simulink model "asbQuadcopters_SiFi"  (Simulink 9.1)
settings: Solver=VariableStepAuto  StartTime=0.0  StopTime=TFinal  RelTol=1e-3
values from neighbouring files (symbols this model uses):
  Controller =     [data_set.mat]
  Estimator =     [data_set.mat]
  g = 9.81    [data_set.mat]
  init =     [data_set.mat]
  rho = 1.184    [data_set.mat]
  sensorCalibrationData = [0.09 -0.06 -9.473 -0.0095 -0.0075 0.0015 101270.95 0.2]    [data_set.mat]
  Sensors =     [data_set.mat]
  States =     [data_set.mat]
  takeOffDuration = 1    [data_set.mat]
  Ts = 0.005    [data_set.mat]
  Vehicle =     [data_set.mat]
undefined symbols (not defined in the file or in its folder): DiscIntNeverNeededParam, Discrete, Earth, ft, m, s, sigbuilder_block, Time, WGS84
libraries: F_Line_block x565, simulink x39, aerolibconvert2 x4, sharedutil x3, ctrlSharedLib x3, sharedtransform x3, shared6dof x1, aerolibasang x1, aerolibtransform2 x1, aerolibnav x1, aerolibanimutils x1
(part 2 of 4)

== system asbQuadcopters_SiFi/Airframe/AC model/Gravity Force Calculation ==
  DCMbe : Inport
  gravity : Inport  Port=2  Unit=m/s^2
  Gain1 : Gain  Gain=Vehicle.Airframe.mass
  FAULT_Gain1 : F_Line_block/Subsystem
  Product : Product  Multiplication=Matrix(*)
  FAULT_Product : F_Line_block/Subsystem
  FAULT_Product_2 : F_Line_block/Subsystem
  gravity force : Outport  Unit=N
  FAULT_gravity force : F_Line_block/Subsystem
  wires:
  gravity/1 -> FAULT_Gain1/1
  FAULT_Gain1/1 -> Gain1/1
  Gain1/1 -> FAULT_Product_2/1  "gravity force NED"
  FAULT_Product_2/1 -> Product/2
  Product/1 -> FAULT_gravity force/1
  FAULT_gravity force/1 -> gravity force/1
  DCMbe/1 -> FAULT_Product/1
  FAULT_Product/1 -> Product/1

== system asbQuadcopters_SiFi/Airframe/AC model/Motor Forces and Torques ==
  Vb : Inport
  Density : Inport  Port=2
  pqr : Inport  Port=3
  Motor  Commands : Inport  Port=4
  D1 : Constant  Value=[Vehicle.Airframe.xy -Vehicle.Airframe.xy Vehicle.Airframe.h]
  D2 : Constant  Value=[Vehicle.Airframe.xy Vehicle.Airframe.xy Vehicle.Airframe.h]
  D3 : Constant  Value=[-Vehicle.Airframe.xy Vehicle.Airframe.xy Vehicle.Airframe.h]
  D4 : Constant  Value=[-Vehicle.Airframe.xy -Vehicle.Airframe.xy Vehicle.Airframe.h]
  For Each Subsystem : Subsystem
  MotorsToW : Subsystem
  Sum of Elements : Sum  Inputs=+  CollapseMode=Specified dimension  CollapseDim=2
  FAULT_Sum of Elements : F_Line_block/Subsystem
  Sum of Elements1 : Sum  Inputs=+  CollapseMode=Specified dimension  CollapseDim=2
  FAULT_Sum of Elements1 : F_Line_block/Subsystem
  Vector Concatenate : Concatenate  NumInputs=4  Mode=Multidimensional array  ConcatenateDimension=2
  FAULT_Vector Concatenate : F_Line_block/Subsystem
  FAULT_Vector Concatenate_2 : F_Line_block/Subsystem
  FAULT_Vector Concatenate_3 : F_Line_block/Subsystem
  FAULT_Vector Concatenate_4 : F_Line_block/Subsystem
  Motor Forces : Outport  Unit=N
  FAULT_Motor Forces : F_Line_block/Subsystem
  Motor Torques : Outport  Port=2  Unit=N*m
  FAULT_Motor Torques : F_Line_block/Subsystem
  wires:
  D2/1 -> FAULT_Vector Concatenate_2/1
  FAULT_Vector Concatenate_2/1 -> Vector Concatenate/2
  D3/1 -> FAULT_Vector Concatenate_3/1
  FAULT_Vector Concatenate_3/1 -> Vector Concatenate/3
  D1/1 -> FAULT_Vector Concatenate/1
  FAULT_Vector Concatenate/1 -> Vector Concatenate/1
  Vector Concatenate/1 -> For Each Subsystem/5(D)
  pqr/1 -> For Each Subsystem/3(Omega)
  For Each Subsystem/2(Moments) -> FAULT_Sum of Elements1/1
  FAULT_Sum of Elements1/1 -> Sum of Elements1/1
  Sum of Elements/1 -> FAULT_Motor Forces/1
  FAULT_Motor Forces/1 -> Motor Forces/1
  Vb/1 -> For Each Subsystem/1(Vb)
  Motor  Commands/1 -> MotorsToW/1(motors_datin)
  For Each Subsystem/1(Forces) -> FAULT_Sum of Elements/1
  FAULT_Sum of Elements/1 -> Sum of Elements/1
  MotorsToW/1(omegas_datout) -> For Each Subsystem/4(w)
  D4/1 -> FAULT_Vector Concatenate_4/1
  FAULT_Vector Concatenate_4/1 -> Vector Concatenate/4
  Density/1 -> For Each Subsystem/2(rho)
  Sum of Elements1/1 -> FAULT_Motor Torques/1
  FAULT_Motor Torques/1 -> Motor Torques/1

== system asbQuadcopters_SiFi/FCS/Crash Predictor Flags/Geofencing error ==
  Action Port : ActionPort  ActionType=then
  FAULT_Action Port : F_Line_block/Subsystem
  Constant : Constant  OutDataTypeStr=uint8
  Out1 : Outport
  FAULT_Out1 : F_Line_block/Subsystem
  wires:
  Constant/1 -> FAULT_Out1/1
  FAULT_Out1/1 -> Out1/1

== system asbQuadcopters_SiFi/FCS/Crash Predictor Flags/Normal condition ==
  Action Port : ActionPort  ActionType=else
  FAULT_Action Port : F_Line_block/Subsystem
  Constant : Constant  Value=0  OutDataTypeStr=uint8
  Out1 : Outport
  FAULT_Out1 : F_Line_block/Subsystem
  wires:
  Constant/1 -> FAULT_Out1/1
  FAULT_Out1/1 -> Out1/1

== system asbQuadcopters_SiFi/FCS/Crash Predictor Flags/estimator/Optical flow error ==
  Action Port : ActionPort  ActionType=elseif
  FAULT_Action Port : F_Line_block/Subsystem
  Constant : Constant  Value=99  OutDataTypeStr=uint8
  Out1 : Outport
  FAULT_Out1 : F_Line_block/Subsystem
  wires:
  Constant/1 -> FAULT_Out1/1
  FAULT_Out1/1 -> Out1/1

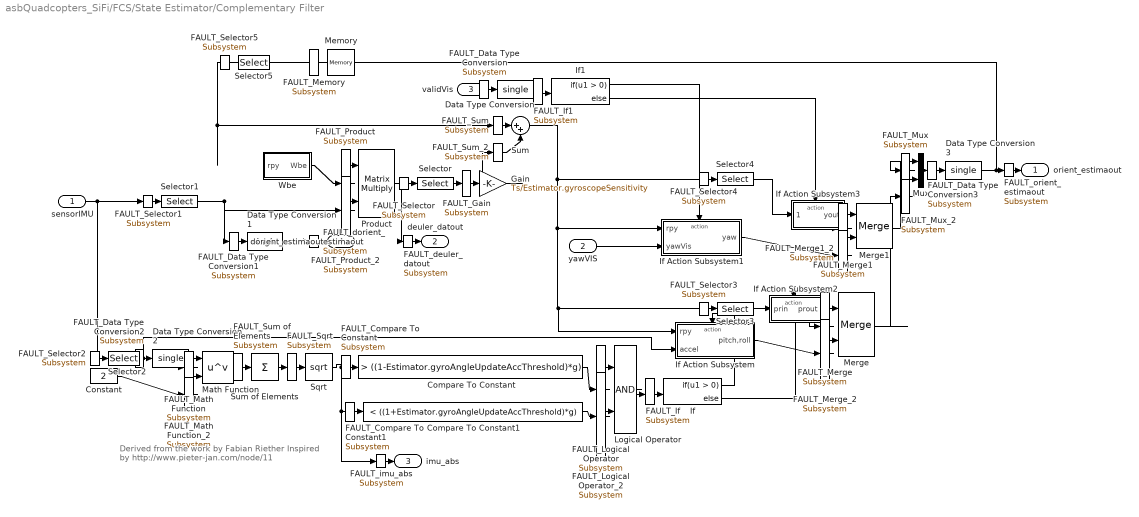
== system asbQuadcopters_SiFi/FCS/State Estimator/Complementary Filter ==
  note: Derived from the work by Fabian Riether
      | Inspired by http://www.pieter-jan.com/node/11
  sensorIMU : Inport  OutDataTypeStr=single
  yawVIS : Inport  Port=2
  validVis : Inport  Port=3
  Compare To Constant : simulink/Logic and Bit Operations/Compare To Constant  relop=>  const=((1-Estimator.gyroAngleUpdateAccThreshold)*g)  OutDataTypeStr=boolean
  FAULT_Compare To Constant : F_Line_block/Subsystem
  Compare To Constant1 : simulink/Logic and Bit Operations/Compare To Constant  relop=<  const=((1+Estimator.gyroAngleUpdateAccThreshold)*g)  OutDataTypeStr=boolean
  FAULT_Compare To Constant1 : F_Line_block/Subsystem
  Constant : Constant  Value=2  OutDataTypeStr=single
  Data Type Conversion{,1..3} (4 alike) : DataTypeConversion  OutDataTypeStr=single
  FAULT_Data Type Conversion{,1..3} (4 alike) : F_Line_block/Subsystem
  Gain : Gain  Gain=Ts/Estimator.gyroscopeSensitivity
  FAULT_Gain : F_Line_block/Subsystem
  If : If
  FAULT_If : F_Line_block/Subsystem
  If Action Subsystem : Subsystem  TreatAsAtomicUnit=on
  If Action Subsystem1 : Subsystem  TreatAsAtomicUnit=on
  If Action Subsystem2 : Subsystem  TreatAsAtomicUnit=on
  If Action Subsystem3 : Subsystem  TreatAsAtomicUnit=on
  If1 : If
  FAULT_If1 : F_Line_block/Subsystem
  Logical Operator : Logic  AllPortsSameDT=off  OutDataTypeStr=fixdt(1,16)
  FAULT_Logical Operator : F_Line_block/Subsystem
  FAULT_Logical Operator_2 : F_Line_block/Subsystem
  Math Function : Math  Operator=pow  SaturateOnIntegerOverflow=on
  FAULT_Math Function : F_Line_block/Subsystem
  FAULT_Math Function_2 : F_Line_block/Subsystem
  Memory : Memory  InitialCondition=single(Estimator.complementaryFilterInit)  InheritSampleTime=on
  FAULT_Memory : F_Line_block/Subsystem
  Merge : Merge
  FAULT_Merge : F_Line_block/Subsystem
  FAULT_Merge_2 : F_Line_block/Subsystem
  Merge1 : Merge
  FAULT_Merge1 : F_Line_block/Subsystem
  FAULT_Merge1_2 : F_Line_block/Subsystem
  Mux : Mux  Inputs=2
  FAULT_Mux : F_Line_block/Subsystem
  FAULT_Mux_2 : F_Line_block/Subsystem
  Product : Product  Multiplication=Matrix(*)
  FAULT_Product : F_Line_block/Subsystem
  FAULT_Product_2 : F_Line_block/Subsystem
  Selector : Selector  InputPortWidth=3  IndexOptions=Index vector (dialog)  Indices=[3 2 1]  OutputSizes=1
  FAULT_Selector{,1..5} (6 alike) : F_Line_block/Subsystem
  Selector1 : Selector  InputPortWidth=6  IndexOptions=Index vector (dialog)  Indices=[4 5 6]  OutputSizes=1
  Selector2 : Selector  InputPortWidth=6  IndexOptions=Index vector (dialog)  Indices=[1 2 3]  OutputSizes=1
  Selector3 : Selector  InputPortWidth=3  IndexOptions=Index vector (dialog)  Indices=[2 1]  OutputSizes=1
  Selector4 : Selector  InputPortWidth=3  IndexOptions=Index vector (dialog)  Indices=[3]  OutputSizes=1
  Selector5 : Selector  InputPortWidth=3  IndexOptions=Index vector (dialog)  Indices=[3 2 1]  OutputSizes=1
  Sqrt : Sqrt  SaturateOnIntegerOverflow=on
  FAULT_Sqrt : F_Line_block/Subsystem
  Sum : Sum  Inputs=|++
  FAULT_Sum : F_Line_block/Subsystem
  FAULT_Sum_2 : F_Line_block/Subsystem
  Sum of Elements : Sum  Inputs=+
  FAULT_Sum of Elements : F_Line_block/Subsystem
  Wbe : Subsystem
  orient_estimaout : Outport
  FAULT_orient_estimaout : F_Line_block/Subsystem
  deuler_datout : Outport  Port=2
  FAULT_deuler_datout : F_Line_block/Subsystem
  imu_abs : Outport  Port=3  OutDataTypeStr=single
  FAULT_imu_abs : F_Line_block/Subsystem
  dorient_estimaout : Outport  Port=4
  FAULT_dorient_estimaout : F_Line_block/Subsystem
  wires:
  sensorIMU/1 -> FAULT_Selector1/1, FAULT_Selector2/1
  FAULT_Selector1/1 -> Selector1/1
  FAULT_Selector2/1 -> Selector2/1
  Product/1 -> FAULT_deuler_datout/1, FAULT_Selector/1
  FAULT_deuler_datout/1 -> deuler_datout/1
  FAULT_Selector/1 -> Selector/1
  Wbe/1(Wbe) -> FAULT_Product/1
  FAULT_Product/1 -> Product/1
  Selector/1 -> FAULT_Gain/1
  FAULT_Gain/1 -> Gain/1
  Gain/1 -> FAULT_Sum_2/1
  FAULT_Sum_2/1 -> Sum/2
  Memory/1 -> FAULT_Selector5/1
  FAULT_Selector5/1 -> Selector5/1
  Sum of Elements/1 -> FAULT_Sqrt/1
  FAULT_Sqrt/1 -> Sqrt/1
  Math Function/1 -> FAULT_Sum of Elements/1
  FAULT_Sum of Elements/1 -> Sum of Elements/1
  Constant/1 -> FAULT_Math Function_2/1
  FAULT_Math Function_2/1 -> Math Function/2
  Selector2/1 -> If Action Subsystem/2(accel), FAULT_Data Type Conversion2/1
  FAULT_deuler_datout/1 -> deuler_datout/1
  FAULT_Data Type Conversion2/1 -> Data Type Conversion2/1
  Sqrt/1 -> FAULT_imu_abs/1, Compare To Constant1/1, Compare To Constant/1
  Compare To Constant/1 -> FAULT_Logical Operator/1
  FAULT_Logical Operator/1 -> Logical Operator/1
  Compare To Constant1/1 -> FAULT_Logical Operator_2/1
  FAULT_Logical Operator_2/1 -> Logical Operator/2
  If Action Subsystem/1(pitch,roll) -> FAULT_Merge_2/1
  FAULT_Merge_2/1 -> Merge/2
  Sum/1 -> If Action Subsystem1/1(rpy), If Action Subsystem/1(rpy), Selector3/1, Selector4/1
  Selector3/1 -> If Action Subsystem2/1(prin)
  yawVIS/1 -> If Action Subsystem1/2(yawVis)
  Selector4/1 -> If Action Subsystem3/1(yawin)
  If Action Subsystem1/1(yaw) -> FAULT_Merge1_2/1
  FAULT_imu_abs/1 -> imu_abs/1
  FAULT_Data Type Conversion2/1 -> Data Type Conversion2/1
  FAULT_Selector2/1 -> Selector2/1
  FAULT_Merge1_2/1 -> Merge1/2
  Merge/1 -> FAULT_Mux_2/1
  FAULT_Mux_2/1 -> Mux/2
  Mux/1 -> FAULT_Data Type Conversion3/1
  FAULT_Data Type Conversion3/1 -> Data Type Conversion3/1
  If Action Subsystem2/1(prout) -> FAULT_Merge/1
  FAULT_Merge/1 -> Merge/1
  If/2 -> If Action Subsystem2/Action
  If Action Subsystem3/1(yout) -> FAULT_Merge1/1
  FAULT_Merge1/1 -> Merge1/1
  If1/2 -> If Action Subsystem3/Action
  Logical Operator/1 -> FAULT_If/1
  FAULT_If/1 -> If/1
  If/1 -> If Action Subsystem/Action
  If1/1 -> If Action Subsystem1/Action
  Data Type Conversion/1 -> FAULT_If1/1
  FAULT_If1/1 -> If1/1
  validVis/1 -> FAULT_Data Type Conversion/1
  FAULT_Data Type Conversion/1 -> Data Type Conversion/1
  Selector1/1 -> FAULT_Product_2/1, FAULT_Data Type Conversion1/1
  FAULT_Product_2/1 -> Product/2
  FAULT_Data Type Conversion1/1 -> Data Type Conversion1/1
  Data Type Conversion2/1 -> FAULT_Math Function/1
  FAULT_Math Function/1 -> Math Function/1
  Data Type Conversion3/1 -> FAULT_Memory/1, FAULT_orient_estimaout/1
  FAULT_Memory/1 -> Memory/1
  FAULT_orient_estimaout/1 -> orient_estimaout/1
  Merge1/1 -> FAULT_Mux/1
  FAULT_Mux/1 -> Mux/1
  Selector5/1 -> FAULT_Sum/1, ?FAULT_Wbe/1
  FAULT_Sum/1 -> Sum/1
  ?FAULT_Wbe/1 -> Wbe/1(rpy)
  Data Type Conversion1/1 -> FAULT_dorient_estimaout/1
  FAULT_dorient_estimaout/1 -> dorient_estimaout/1

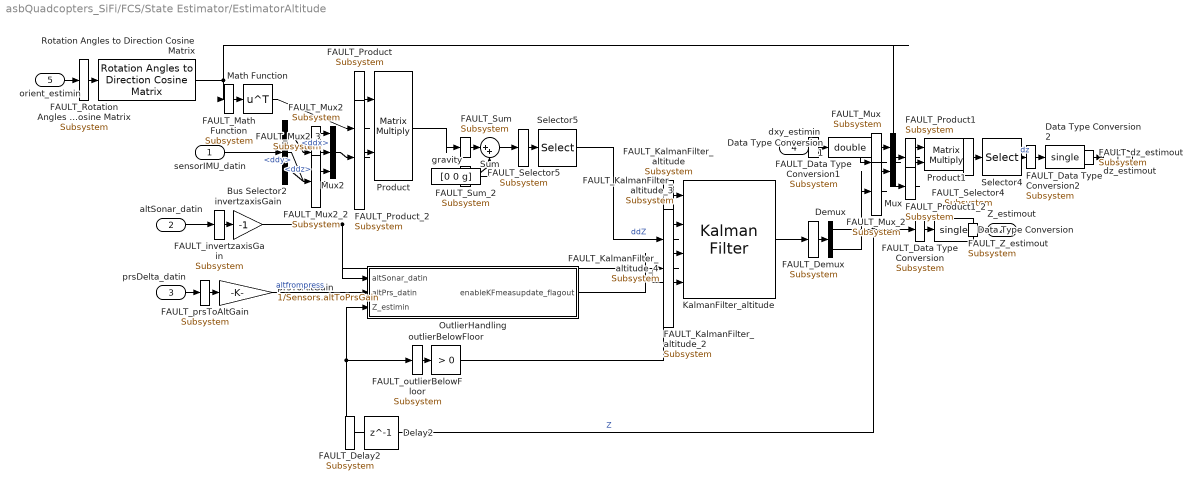
== system asbQuadcopters_SiFi/FCS/State Estimator/EstimatorAltitude ==
  sensorIMU_datin : Inport
  altSonar_datin : Inport  Port=2
  prsDelta_datin : Inport  Port=3
  dxy_estimin : Inport  Port=4
  orient_estimin : Inport  Port=5
  Bus Selector2 : BusSelector  OutputSignals=ddx,ddy,ddz
  Data Type Conversion : DataTypeConversion  OutDataTypeStr=single  SaturateOnIntegerOverflow=on
  FAULT_Data Type Conversion : F_Line_block/Subsystem
  Data Type Conversion1 : DataTypeConversion  OutDataTypeStr=double  SaturateOnIntegerOverflow=on
  FAULT_Data Type Conversion1 : F_Line_block/Subsystem
  Data Type Conversion2 : DataTypeConversion  OutDataTypeStr=single  SaturateOnIntegerOverflow=on
  FAULT_Data Type Conversion2 : F_Line_block/Subsystem
  Delay2 : Delay  DelayLength=1  InitialCondition=0
  FAULT_Delay2 : F_Line_block/Subsystem
  Demux : Demux  Outputs=2
  FAULT_Demux : F_Line_block/Subsystem
  KalmanFilter_altitude : ctrlSharedLib/Kalman Filter  TimeDomain=Discrete-Time  UseCurrentEstimator=on  ModelSource=Individual A, B, C, D matrices  ModelSourceVariable=sys  A=[1 Ts; 0 1]  B=[0;Ts]  C=[1 0]  D=[0]  NumberOfStates=2  NumberOfInputs=2  NumberOfOutputs=2  InitialEstimateSource=Dialog  X0=[init.posNED(3) 0]  P0=10  UseK=off  UseGH=on  NumberOfProcessNoiseInputs=2  G=Estimator.alt.kf.G  TimeInvariantG=on  H=Estimator.alt.kf.H  TimeInvariantH=on  Q=Estimator.alt.kf.Q  TimeInvariantQ=on  R=Estimator.alt.kf.R  TimeInvariantR=on  N=Estimator.alt.kf.N  TimeInvariantN=on  AddInputPort=on  AddEnablePort=on  ExternalReset=Level hold  OutputEstimatedY=off  OutputP=off  Ts=-1
      settings: SourceProductBaseCode=CT
  FAULT_KalmanFilter_altitude : F_Line_block/Subsystem
  FAULT_KalmanFilter_altitude_2 : F_Line_block/Subsystem
  FAULT_KalmanFilter_altitude_3 : F_Line_block/Subsystem
  FAULT_KalmanFilter_altitude_4 : F_Line_block/Subsystem
  Math Function : Math  Operator=transpose  SaturateOnIntegerOverflow=on
  FAULT_Math Function : F_Line_block/Subsystem
  Mux : Mux  Inputs=2
  FAULT_Mux : F_Line_block/Subsystem
  FAULT_Mux_2 : F_Line_block/Subsystem
  Mux2 : Mux  Inputs=3
  FAULT_Mux2 : F_Line_block/Subsystem
  FAULT_Mux2_2 : F_Line_block/Subsystem
  FAULT_Mux2_3 : F_Line_block/Subsystem
  OutlierHandling : Subsystem
  Product : Product  Multiplication=Matrix(*)
  FAULT_Product : F_Line_block/Subsystem
  FAULT_Product_2 : F_Line_block/Subsystem
  Product1 : Product  Multiplication=Matrix(*)
  FAULT_Product1 : F_Line_block/Subsystem
  FAULT_Product1_2 : F_Line_block/Subsystem
  Rotation Angles to Direction Cosine Matrix : sharedtransform/Rotation Angles to Direction Cosine Matrix  rotationOrder=ZYX  aMode=aMode
      settings: SourceProductBaseCode=AE
  FAULT_Rotation Angles to Direction Cosine Matrix : F_Line_block/Subsystem
  Selector4 : Selector  InputPortWidth=3  IndexOptions=Index vector (dialog)  Indices=[3]  OutputSizes=1
  FAULT_Selector4 : F_Line_block/Subsystem
  Selector5 : Selector  InputPortWidth=3  IndexOptions=Index vector (dialog)  Indices=[3]  OutputSizes=1
  FAULT_Selector5 : F_Line_block/Subsystem
  Sum : Sum  Inputs=|++
  FAULT_Sum : F_Line_block/Subsystem
  FAULT_Sum_2 : F_Line_block/Subsystem
  gravity : Constant  Value=[0 0 g]
  invertzaxisGain : Gain  Gain=-1  ParamDataTypeStr=single  OutDataTypeStr=double
  FAULT_invertzaxisGain : F_Line_block/Subsystem
  outlierBelowFloor : simulink/Logic and Bit Operations/Compare To Constant  relop=>  const=0  OutDataTypeStr=boolean
  FAULT_outlierBelowFloor : F_Line_block/Subsystem
  prsToAltGain : Gain  Gain=1/Sensors.altToPrsGain
  FAULT_prsToAltGain : F_Line_block/Subsystem
  dz_estimout : Outport
  FAULT_dz_estimout : F_Line_block/Subsystem
  Z_estimout : Outport  Port=2
  FAULT_Z_estimout : F_Line_block/Subsystem
  wires:
  Mux2/1 -> FAULT_Product_2/1
  FAULT_Product_2/1 -> Product/2
  sensorIMU_datin/1 -> Bus Selector2/1
  Bus Selector2/3 -> FAULT_Mux2_3/1  "<ddz>"
  FAULT_Mux2_3/1 -> Mux2/3
  Bus Selector2/2 -> FAULT_Mux2_2/1  "<ddy>"
  FAULT_Mux2_2/1 -> Mux2/2
  Bus Selector2/1 -> FAULT_Mux2/1  "<ddx>"
  FAULT_Mux2/1 -> Mux2/1
  Product1/1 -> FAULT_Selector4/1
  FAULT_Selector4/1 -> Selector4/1
  dxy_estimin/1 -> FAULT_Data Type Conversion1/1
  FAULT_Data Type Conversion1/1 -> Data Type Conversion1/1
  Delay2/1 -> OutlierHandling/3(Z_estimin), FAULT_outlierBelowFloor/1
  ?FAULT_Add1/1 -> ?Add1/1
  FAULT_outlierBelowFloor/1 -> outlierBelowFloor/1
  prsToAltGain/1 -> OutlierHandling/2(altPrs_datin)  "altfrompress"
  prsDelta_datin/1 -> FAULT_prsToAltGain/1
  FAULT_prsToAltGain/1 -> prsToAltGain/1
  outlierBelowFloor/1 -> FAULT_KalmanFilter_altitude_4/1
  FAULT_KalmanFilter_altitude_4/1 -> KalmanFilter_altitude/4
  Demux/2 -> FAULT_Mux_2/1
  FAULT_Mux_2/1 -> Mux/2
  Selector4/1 -> FAULT_Data Type Conversion2/1  "dz"
  FAULT_Data Type Conversion2/1 -> Data Type Conversion2/1
  Demux/1 -> FAULT_Data Type Conversion/1, FAULT_Delay2/1  "Z"
  FAULT_Data Type Conversion/1 -> Data Type Conversion/1
  FAULT_Delay2/1 -> Delay2/1
  Selector5/1 -> FAULT_KalmanFilter_altitude/1  "ddZ"
  FAULT_KalmanFilter_altitude/1 -> KalmanFilter_altitude/1
  Mux/1 -> FAULT_Product1_2/1
  FAULT_Product1_2/1 -> Product1/2
  KalmanFilter_altitude/1 -> FAULT_Demux/1
  FAULT_Demux/1 -> Demux/1
  Sum/1 -> FAULT_Selector5/1
  FAULT_Selector5/1 -> Selector5/1
  gravity/1 -> FAULT_Sum_2/1
  FAULT_Sum_2/1 -> Sum/2
  Product/1 -> FAULT_Sum/1
  FAULT_Sum/1 -> Sum/1
  altSonar_datin/1 -> FAULT_invertzaxisGain/1
  FAULT_invertzaxisGain/1 -> invertzaxisGain/1
  orient_estimin/1 -> FAULT_Rotation Angles to Direction Cosine Matrix/1
  FAULT_Rotation Angles to Direction Cosine Matrix/1 -> Rotation Angles to Direction Cosine Matrix/1
  Data Type Conversion/1 -> FAULT_Z_estimout/1
  FAULT_Z_estimout/1 -> Z_estimout/1
  Data Type Conversion1/1 -> FAULT_Mux/1
  FAULT_Mux/1 -> Mux/1
  Math Function/1 -> FAULT_Product/1
  FAULT_Product/1 -> Product/1
  invertzaxisGain/1 -> FAULT_KalmanFilter_altitude_2/1, OutlierHandling/1(altSonar_datin)
  FAULT_KalmanFilter_altitude_2/1 -> KalmanFilter_altitude/2
  FAULT_Delay2/1 -> Delay2/1
  Data Type Conversion2/1 -> FAULT_dz_estimout/1
  FAULT_dz_estimout/1 -> dz_estimout/1
  OutlierHandling/1(enableKFmeasupdate_flagout) -> FAULT_KalmanFilter_altitude_3/1
  FAULT_KalmanFilter_altitude_3/1 -> KalmanFilter_altitude/3
  Rotation Angles to Direction Cosine Matrix/1 -> FAULT_Math Function/1, FAULT_Product1/1
  FAULT_Math Function/1 -> Math Function/1
  FAULT_Product1/1 -> Product1/1

== system asbQuadcopters_SiFi/FCS/State Estimator/EstimatorXYPosition ==
  opticalFlow_datin : Inport
  controlModePosVSOrient_flagin : Inport  Port=2
  usePosVIS_flagin : Inport  Port=3
  posVIS_datin : Inport  Port=4
  sensorIMU_datin : Inport  Port=5
  Z_estimin : Inport  Port=6
  dz_estimin : Inport  Port=7
  orient_estimin : Inport  Port=8
  EstimatorVelocity : Subsystem
  EstimatorXYPosition : Subsystem
  XY_estimout : Outport
  FAULT_XY_estimout : F_Line_block/Subsystem
  dxy_estimout : Outport  Port=2
  FAULT_dxy_estimout : F_Line_block/Subsystem
  wires:
  EstimatorXYPosition/1(XY_estimout) -> FAULT_XY_estimout/1
  FAULT_XY_estimout/1 -> XY_estimout/1
  usePosVIS_flagin/1 -> EstimatorXYPosition/6(usePosVIS_flagin)
  posVIS_datin/1 -> EstimatorXYPosition/5(posVIS_datin)
  dz_estimin/1 -> EstimatorXYPosition/4(dz_estimin)
  controlModePosVSOrient_flagin/1 -> EstimatorXYPosition/3(controlModePosVSOrient_flagin)
  Z_estimin/1 -> EstimatorVelocity/2(Z_estimin)
  sensorIMU_datin/1 -> EstimatorVelocity/3(sensorIMU_datin)
  opticalFlow_datin/1 -> EstimatorVelocity/1(opticalFlow_datin)
  EstimatorVelocity/1(dxy_estimout) -> FAULT_dxy_estimout/1, EstimatorXYPosition/1(dxy_estimin)
  FAULT_dxy_estimout/1 -> dxy_estimout/1
  ?FAULT_KalmanFilter_posxy/1 -> ?KalmanFilter_posxy/1
  orient_estimin/1 -> EstimatorXYPosition/2(orient_estimin), EstimatorVelocity/4(orient_estimin)

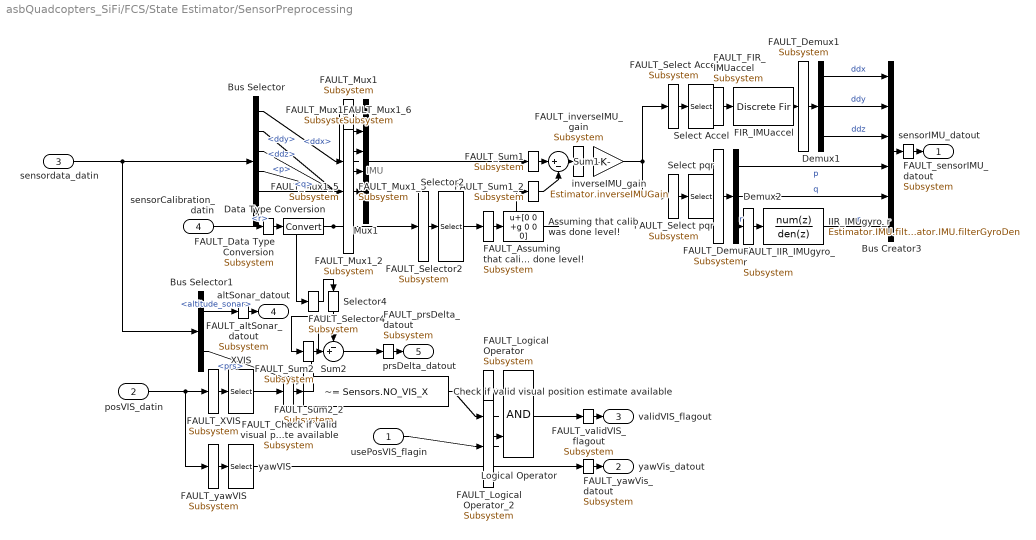
== system asbQuadcopters_SiFi/FCS/State Estimator/SensorPreprocessing ==
  note: IMU
  usePosVIS_flagin : Inport
  posVIS_datin : Inport  Port=2
  sensordata_datin : Inport  Port=3
  sensorCalibration_datin : Inport  Port=4
  Assuming that calib was done level! : Bias  Bias=[0 0 +g 0 0 0]
  FAULT_Assuming that calib was done level! : F_Line_block/Subsystem
  Bus Creator3 : BusCreator  Inputs=6
  Bus Selector : BusSelector  OutputSignals=ddx,ddy,ddz,p,q,r
  Bus Selector1 : BusSelector  OutputSignals=altitude_sonar,prs
  Check if valid visual position estimate available : simulink/Logic and Bit Operations/Compare To Constant  relop=~=  const=Sensors.NO_VIS_X  OutDataTypeStr=boolean
  FAULT_Check if valid visual position estimate available : F_Line_block/Subsystem
  Data Type Conversion : DataTypeConversion
  FAULT_Data Type Conversion : F_Line_block/Subsystem
  Demux1 : Demux  Outputs=3
  FAULT_Demux1 : F_Line_block/Subsystem
  Demux2 : Demux  Outputs=3
  FAULT_Demux2 : F_Line_block/Subsystem
  FIR_IMUaccel : DiscreteFir  Coefficients=Estimator.IMU.filterAccel.Coefficients
  FAULT_FIR_IMUaccel : F_Line_block/Subsystem
  IIR_IMUgyro_r : DiscreteFilter  Numerator=Estimator.IMU.filterGyroNum  Denominator=Estimator.IMU.filterGyroDen
  FAULT_IIR_IMUgyro_r : F_Line_block/Subsystem
  Logical Operator : Logic  AllPortsSameDT=off  OutDataTypeStr=boolean
  FAULT_Logical Operator : F_Line_block/Subsystem
  FAULT_Logical Operator_2 : F_Line_block/Subsystem
  Mux1 : Mux  Inputs=6
  FAULT_Mux1 : F_Line_block/Subsystem
  FAULT_Mux1_{2..6} (5 alike) : F_Line_block/Subsystem
  Select Accel : Selector  InputPortWidth=6  IndexOptions=Index vector (dialog)  Indices=[1 2 3]  OutputSizes=1
  FAULT_Select Accel : F_Line_block/Subsystem
  Select pqr : Selector  InputPortWidth=6  IndexOptions=Index vector (dialog)  Indices=[4 5 6]  OutputSizes=1
  FAULT_Select pqr : F_Line_block/Subsystem
  Selector2 : Selector  InputPortWidth=8  IndexOptions=Index vector (dialog)  Indices=[1:6]  OutputSizes=1
  FAULT_Selector2 : F_Line_block/Subsystem
  Selector4 : Selector  InputPortWidth=8  IndexOptions=Index vector (dialog)  Indices=[7]  OutputSizes=1
  FAULT_Selector4 : F_Line_block/Subsystem
  Sum1 : Sum  Inputs=|+-
  FAULT_Sum1 : F_Line_block/Subsystem
  FAULT_Sum1_2 : F_Line_block/Subsystem
  Sum2 : Sum  Inputs=-+|
  FAULT_Sum2 : F_Line_block/Subsystem
  FAULT_Sum2_2 : F_Line_block/Subsystem
  XVIS : Selector  InputPortWidth=4  IndexOptions=Index vector (dialog)  Indices=1  OutputSizes=1
  FAULT_XVIS : F_Line_block/Subsystem
  inverseIMU_gain : Gain  Gain=Estimator.inverseIMUGain  ParamDataTypeStr=single  OutDataTypeStr=single
  FAULT_inverseIMU_gain : F_Line_block/Subsystem
  yawVIS : Selector  InputPortWidth=4  IndexOptions=Index vector (dialog)  Indices=4  OutputSizes=1
  FAULT_yawVIS : F_Line_block/Subsystem
  sensorIMU_datout : Outport
  FAULT_sensorIMU_datout : F_Line_block/Subsystem
  yawVis_datout : Outport  Port=2
  FAULT_yawVis_datout : F_Line_block/Subsystem
  validVIS_flagout : Outport  Port=3
  FAULT_validVIS_flagout : F_Line_block/Subsystem
  altSonar_datout : Outport  Port=4
  FAULT_altSonar_datout : F_Line_block/Subsystem
  prsDelta_datout : Outport  Port=5
  FAULT_prsDelta_datout : F_Line_block/Subsystem
  wires:
  Select pqr/1 -> FAULT_Demux2/1
  ?FAULT_dxy_estimout/1 -> ?dxy_estimout/1
  ?FAULT_KalmanFilter_posxy/1 -> ?KalmanFilter_posxy/1
  FAULT_Demux2/1 -> Demux2/1
  Assuming that calib was done level!/1 -> FAULT_Sum1_2/1
  FAULT_Sum1_2/1 -> Sum1/2
  usePosVIS_flagin/1 -> FAULT_Logical Operator_2/1
  FAULT_Logical Operator_2/1 -> Logical Operator/2
  Check if valid visual position estimate available/1 -> FAULT_Logical Operator/1
  FAULT_Logical Operator/1 -> Logical Operator/1
  Logical Operator/1 -> FAULT_validVIS_flagout/1
  FAULT_validVIS_flagout/1 -> validVIS_flagout/1
  yawVIS/1 -> FAULT_yawVis_datout/1
  FAULT_yawVis_datout/1 -> yawVis_datout/1
  XVIS/1 -> FAULT_Check if valid visual position estimate available/1
  FAULT_Check if valid visual position estimate available/1 -> Check if valid visual position estimate available/1
  Mux1/1 -> FAULT_Sum1/1
  FAULT_Sum1/1 -> Sum1/1
  Sum2/1 -> FAULT_prsDelta_datout/1
  FAULT_prsDelta_datout/1 -> prsDelta_datout/1
  Bus Selector1/2 -> FAULT_Sum2_2/1  "<prs>"
  FAULT_Sum2_2/1 -> Sum2/2
  Selector4/1 -> FAULT_Sum2/1
  FAULT_Sum2/1 -> Sum2/1
  Bus Selector1/1 -> FAULT_altSonar_datout/1  "<altitude_sonar>"
  FAULT_altSonar_datout/1 -> altSonar_datout/1
  sensordata_datin/1 -> Bus Selector1/1, Bus Selector/1
  Bus Selector/6 -> ?  "<r>"
  ?FAULT_dxy_estimout/1 -> ?dxy_estimout/1
  ?FAULT_KalmanFilter_posxy/1 -> ?KalmanFilter_posxy/1
  FAULT_Mux1/1 -> Mux1/1
  Bus Selector/5 -> FAULT_Mux1_5/1  "<q>"
  FAULT_Mux1_5/1 -> Mux1/5
  Bus Selector/4 -> FAULT_Mux1_4/1  "<p>"
  FAULT_Mux1_4/1 -> Mux1/4
  Bus Selector/3 -> FAULT_Mux1_3/1  "<ddz>"
  FAULT_Mux1_3/1 -> Mux1/3
  Bus Selector/2 -> FAULT_Mux1_2/1  "<ddy>"
  FAULT_Mux1_2/1 -> Mux1/2
  Bus Selector/1 -> FAULT_Mux1/1  "<ddx>"
  FAULT_Mux1/1 -> Mux1/1
  sensorCalibration_datin/1 -> FAULT_Data Type Conversion/1
  FAULT_Data Type Conversion/1 -> Data Type Conversion/1
  IIR_IMUgyro_r/1 -> Bus Creator3/6  "r"
  Demux2/3 -> FAULT_IIR_IMUgyro_r/1  "r"
  FAULT_IIR_IMUgyro_r/1 -> IIR_IMUgyro_r/1
  FIR_IMUaccel/1 -> FAULT_Demux1/1
  FAULT_Demux1/1 -> Demux1/1
  Select Accel/1 -> FAULT_FIR_IMUaccel/1
  FAULT_FIR_IMUaccel/1 -> FIR_IMUaccel/1
  inverseIMU_gain/1 -> FAULT_Select Accel/1, FAULT_Select pqr/1
  FAULT_Select Accel/1 -> Select Accel/1
  FAULT_Select pqr/1 -> Select pqr/1
  Demux2/2 -> Bus Creator3/5  "q"
  Demux2/1 -> Bus Creator3/4  "p"
  Selector2/1 -> FAULT_Assuming that calib was done level!/1
  FAULT_Assuming that calib was done level!/1 -> Assuming that calib was done level!/1
  Sum1/1 -> FAULT_inverseIMU_gain/1
  FAULT_inverseIMU_gain/1 -> inverseIMU_gain/1
  Demux1/3 -> Bus Creator3/3  "ddz"
  Demux1/2 -> Bus Creator3/2  "ddy"
  Demux1/1 -> Bus Creator3/1  "ddx"
  Bus Creator3/1 -> FAULT_sensorIMU_datout/1
  FAULT_sensorIMU_datout/1 -> sensorIMU_datout/1
  posVIS_datin/1 -> FAULT_XVIS/1, FAULT_yawVIS/1
  FAULT_XVIS/1 -> XVIS/1
  FAULT_yawVIS/1 -> yawVIS/1
  Data Type Conversion/1 -> FAULT_Selector2/1, FAULT_Selector4/1
  FAULT_Selector2/1 -> Selector2/1
  FAULT_Selector4/1 -> Selector4/1

== system asbQuadcopters_SiFi/FCS/controller/Attitude ==
  note: ATTITUDE
  refAttitude : Inport
  states_estim : Inport  Port=2
  Add : Sum  Inputs=+-
  Bus Selector3 : BusSelector  OutputSignals=pitch,roll
  Bus Selector4 : BusSelector  OutputSignals=q,p
  D_pr : Gain  Gain=[0.002;0.003]
  Delay : Delay  DelayLength=1  InitialCondition=0
  Demux : Demux  Outputs=2
  Discrete-Time Integrator : DiscreteIntegrator  SampleTime=Ts  LimitOutput=on  UpperSaturationLimit=2  LowerSaturationLimit=-2  ICPrevOutput=DiscIntNeverNeededParam  ICPrevScaledInput=DiscIntNeverNeededParam
  I_pr : Gain  Gain=0.01
  Mux : Mux  Inputs=2
  Mux1 : Mux  Inputs=2
  P_pr : Gain  Gain=[0.013;0.02]
  Sum16 : Sum  Inputs=++-  AccumDataTypeStr=single  OutDataTypeStr=single  SaturateOnIntegerOverflow=on
  Sum19 : Sum  Inputs=+-|
  antiWU_Gain : Gain  Gain=0.001
  tau_pitch : Outport
  tau_roll : Outport  Port=2
  wires:
  Sum16/1 -> Demux/1  "P_pr"
  antiWU_Gain/1 -> Add/2
  Add/1 -> Discrete-Time Integrator/1
  Bus Selector3/1 -> Mux/1  "<pitch>"
  Bus Selector4/1 -> Mux1/1  "<q>"
  P_pr/1 -> Sum16/1
  I_pr/1 -> Sum16/2
  Sum19/1 -> Add/1, P_pr/1  "pitch/roll error"
  Discrete-Time Integrator/1 -> Delay/1, I_pr/1
  Delay/1 -> antiWU_Gain/1
  Demux/1 -> tau_pitch/1  "tau_pitch"
  Demux/2 -> tau_roll/1
  D_pr/1 -> Sum16/3
  states_estim/1 -> Bus Selector3/1, Bus Selector4/1
  refAttitude/1 -> Sum19/1
  Mux/1 -> Sum19/2
  Bus Selector3/2 -> Mux/2  "<roll>"
  Mux1/1 -> D_pr/1
  Bus Selector4/2 -> Mux1/2  "<p>"

== system asbQuadcopters_SiFi/FCS/controller/ControlMixer ==
  tau_pitch : Inport
  tau_roll : Inport  Port=2
  tau_yaw : Inport  Port=3
  totalThrust : Inport  Port=4
  Mux2 : Mux
  Product : Product  Multiplication=Matrix(*)  RndMeth=Zero
  TorqueTotalThrustToThrustPerMotor : Constant  Value=Controller.Q2Ts  OutDataTypeStr=single
  thrusts_refout : Outport
  wires:
  Product/1 -> ?FAULT_thrusts_refout/1
  ?FAULT_thrusts_refout/1 -> thrusts_refout/1
  tau_roll/1 -> ?FAULT_Mux2_4/1
  ?FAULT_Mux2_4/1 -> Mux2/4
  tau_pitch/1 -> ?FAULT_Mux2_3/1
  ?FAULT_Mux2_3/1 -> Mux2/3
  tau_yaw/1 -> ?FAULT_Mux2_2/1
  ?FAULT_Mux2_2/1 -> Mux2/2
  totalThrust/1 -> ?FAULT_Mux2/1
  ?FAULT_Mux2/1 -> Mux2/1
  TorqueTotalThrustToThrustPerMotor/1 -> ?FAULT_Product/1
  ?FAULT_Product/1 -> Product/1
  Mux2/1 -> ?FAULT_Product_2/1
  ?FAULT_Product_2/1 -> Product/2

== system asbQuadcopters_SiFi/FCS/controller/XY-to-reference-orientation ==
  posXY : Inport
  states_estim : Inport  Port=2
  yaw : Inport  Port=3
  Bus Selector1 : BusSelector  OutputSignals=X,Y
  Bus Selector2 : BusSelector  OutputSignals=dx,dy
  D_xy : Gain  Gain=[0.1, -0.1]  ParamDataTypeStr=single  OutDataTypeStr=single  SaturateOnIntegerOverflow=on
  Gain : Gain  Gain=-1
  Matrix Concatenate : Concatenate  Mode=Multidimensional array  ConcatenateDimension=2
  Mux : Mux  Inputs=2
  Mux1 : Mux  Inputs=2
  P_xy : Gain  Gain=[-0.24,0.24]  ParamDataTypeStr=single  OutDataTypeStr=single  SaturateOnIntegerOverflow=on
  Product : Product  Multiplication=Matrix(*)  OutDataTypeStr=single  RndMeth=Zero
  Saturation : Saturate  UpperLimit=3  LowerLimit=-3  OutDataTypeStr=single
  Sum17 : Sum  Inputs=+-|  AccumDataTypeStr=single
  Sum18 : Sum  Inputs=|++  AccumDataTypeStr=single  OutDataTypeStr=single  SaturateOnIntegerOverflow=on
  Trigonometric Function : Trigonometry  Operator=sincos
  Vector Concatenate : Concatenate
  Vector Concatenate1 : Concatenate
  pitch_roll_cmd : Outport
  wires:
  yaw/1 -> ?FAULT_Trigonometric Function/1
  ?FAULT_Trigonometric Function/1 -> Trigonometric Function/1
  Saturation/1 -> ?FAULT_P_xy/1
  ?FAULT_P_xy/1 -> P_xy/1
  P_xy/1 -> ?FAULT_Sum18/1
  ?FAULT_Sum18/1 -> Sum18/1
  Sum17/1 -> ?FAULT_Product_2/1  "XY error"
  ?FAULT_Product_2/1 -> Product/2
  posXY/1 -> ?FAULT_Sum17/1
  ?FAULT_Sum17/1 -> Sum17/1
  Bus Selector2/1 -> ?FAULT_Mux1/1  "<dx>"
  ?FAULT_Mux1/1 -> Mux1/1
  states_estim/1 -> Bus Selector1/1, Bus Selector2/1
  Sum18/1 -> ?FAULT_pitch_roll_cmd/1  "pitch/roll cmd"
  ?FAULT_Selector2/1 -> ?Selector2/1
  ?FAULT_Selector4/1 -> ?Selector4/1
  ?FAULT_pitch_roll_cmd/1 -> pitch_roll_cmd/1
  D_xy/1 -> ?FAULT_Sum18_2/1
  ?FAULT_Sum18_2/1 -> Sum18/2
  Bus Selector1/1 -> ?FAULT_Mux/1  "<X>"
  ?FAULT_Mux/1 -> Mux/1
  Product/1 -> ?FAULT_Saturation/1
  ?FAULT_Saturation/1 -> Saturation/1
  Trigonometric Function/1 -> ?FAULT_Gain/1, ?FAULT_Vector Concatenate1/1
  ?FAULT_Gain/1 -> Gain/1
  ?FAULT_Vector Concatenate1/1 -> Vector Concatenate1/1
  Trigonometric Function/2 -> ?FAULT_Vector Concatenate1_2/1, ?FAULT_Vector Concatenate/1
  ?FAULT_Vector Concatenate1_2/1 -> Vector Concatenate1/2
  ?FAULT_Vector Concatenate/1 -> Vector Concatenate/1
  Gain/1 -> ?FAULT_Vector Concatenate_2/1
  ?FAULT_Vector Concatenate_2/1 -> Vector Concatenate/2
  Vector Concatenate/1 -> ?FAULT_Matrix Concatenate/1
  ?FAULT_Matrix Concatenate/1 -> Matrix Concatenate/1
  Vector Concatenate1/1 -> ?FAULT_Matrix Concatenate_2/1
  ?FAULT_Matrix Concatenate_2/1 -> Matrix Concatenate/2
  Matrix Concatenate/1 -> ?FAULT_Product/1
  ?FAULT_Product/1 -> Product/1
  Bus Selector1/2 -> ?FAULT_Mux_2/1  "<Y>"
  ?FAULT_Mux_2/1 -> Mux/2
  Mux/1 -> ?FAULT_Sum17_2/1
  ?FAULT_Sum17_2/1 -> Sum17/2
  Mux1/1 -> ?FAULT_D_xy/1
  ?FAULT_D_xy/1 -> D_xy/1
  Bus Selector2/2 -> ?FAULT_Mux1_2/1  "<dy>"
  ?FAULT_Mux1_2/1 -> Mux1/2

== system asbQuadcopters_SiFi/FCS/controller/Yaw ==
  yaw_ref : Inport
  states_estim : Inport  Port=2
  Bus Selector5 : BusSelector  OutputSignals=yaw,r
  D_yaw : Gain  Gain=0.3*0.004
  P_yaw : Gain  Gain=0.004  ParamDataTypeStr=single  OutDataTypeStr=single
  Sum1 : Sum  Inputs=+-|  AccumDataTypeStr=single  OutDataTypeStr=single  SaturateOnIntegerOverflow=on
  Sum2 : Sum  Inputs=|+-
  yaw : Outport
  tau_yaw : Outport  Port=2
  wires:
  D_yaw/1 -> ?FAULT_Sum2_2/1
  ?FAULT_Sum2_2/1 -> Sum2/2
  P_yaw/1 -> ?FAULT_Sum2/1
  ?FAULT_Sum2/1 -> Sum2/1
  Bus Selector5/2 -> ?FAULT_D_yaw/1  "<r>"
  ?FAULT_D_yaw/1 -> D_yaw/1
  Sum1/1 -> ?FAULT_P_yaw/1
  ?FAULT_P_yaw/1 -> P_yaw/1
  states_estim/1 -> Bus Selector5/1
  Sum2/1 -> ?FAULT_tau_yaw/1
  ?FAULT_tau_yaw/1 -> tau_yaw/1
  Bus Selector5/1 -> ?FAULT_yaw/1, ?FAULT_Sum1_2/1  "<yaw>"
  ?FAULT_yaw/1 -> yaw/1
  ?FAULT_Sum1_2/1 -> Sum1/2
  yaw_ref/1 -> ?FAULT_Sum1/1
  ?FAULT_Sum1/1 -> Sum1/1

== system asbQuadcopters_SiFi/FCS/controller/gravity feedforward/equilibrium thrust ==
  note: ALTITUDE
  states_estim : Inport
  PosZ : Inport  Port=2
  takeoff_flag : Inport  Port=3
  Bus Selector6 : BusSelector  OutputSignals=Z,dz
  D_z : Gain  Gain=0.3  ParamDataTypeStr=single  OutDataTypeStr=single  SaturateOnIntegerOverflow=on
  P_z : Gain  Gain=0.8  ParamDataTypeStr=single  OutDataTypeStr=single  SaturateOnIntegerOverflow=on
  SaturationThrust : Saturate  UpperLimit=4*Controller.totalThrustMaxRelative*Controller.motorsThrustPerMotorMax  LowerLimit=-4*Controller.totalThrustMaxRelative*Controller.motorsThrustPerMotorMax  OutDataTypeStr=single
  Sum15 : Sum  Inputs=|+-  AccumDataTypeStr=single  OutDataTypeStr=single  SaturateOnIntegerOverflow=on
  Sum3 : Sum  Inputs=+-|  AccumDataTypeStr=single  OutDataTypeStr=single  SaturateOnIntegerOverflow=on
  Sum4 : Sum  Inputs=++|  AccumDataTypeStr=single  OutDataTypeStr=single  SaturateOnIntegerOverflow=on
  TakeoffOrControl_Switch : Switch  Criteria=u2 > Threshold
  takeoff_gain : Gain  Gain=Controller.takeoffGain  ParamDataTypeStr=single  OutDataTypeStr=single  SaturateOnIntegerOverflow=on
  w0 : Constant  Value=-g*Vehicle.Airframe.mass  OutDataTypeStr=single  SampleTime=Ts
  altitude_cmd : Outport
  wires:
  Sum3/1 -> ?FAULT_P_z/1  "errZ"
  ?FAULT_P_z/1 -> P_z/1
  TakeoffOrControl_Switch/1 -> ?FAULT_Sum4_2/1
  ?FAULT_Sum4_2/1 -> Sum4/2
  Bus Selector6/1 -> ?FAULT_Sum3_2/1  "<Z>"
  ?FAULT_Sum3_2/1 -> Sum3/2
  Bus Selector6/2 -> ?FAULT_D_z/1  "<dz>"
  ?FAULT_D_z/1 -> D_z/1
  w0/1 -> ?FAULT_Sum4/1, ?FAULT_takeoff_gain/1
  ?FAULT_Sum4/1 -> Sum4/1
  ?FAULT_takeoff_gain/1 -> takeoff_gain/1
  D_z/1 -> ?FAULT_Sum15_2/1  "dz"
  ?FAULT_Sum15_2/1 -> Sum15/2
  takeoff_gain/1 -> TakeoffOrControl_Switch/1
  takeoff_flag/1 -> TakeoffOrControl_Switch/2
  PosZ/1 -> ?FAULT_Sum3/1
  ?FAULT_Sum3/1 -> Sum3/1
  P_z/1 -> ?FAULT_Sum15/1
  ?FAULT_Sum15/1 -> Sum15/1
  Sum15/1 -> TakeoffOrControl_Switch/3
  Sum4/1 -> ?FAULT_SaturationThrust/1
  ?FAULT_SaturationThrust/1 -> SaturationThrust/1
  SaturationThrust/1 -> ?FAULT_altitude_cmd/1
  ?FAULT_altitude_cmd/1 -> altitude_cmd/1
  states_estim/1 -> Bus Selector6/1

== system asbQuadcopters_SiFi/FCS/controller/thrustsToMotorCommands ==
  thrusts_refin : Inport
  MotorDirections : Gain  Gain=[1 -1 1 -1]
  Saturation5 : Saturate  UpperLimit=Vehicle.Motor.maxLimit  LowerLimit=Vehicle.Motor.minLimit
  ThrustToMotorCommand : Gain  Gain=-Vehicle.Motor.thrustToMotorCommand
  motors_cmdout : Outport
  wires:
  Saturation5/1 -> MotorDirections/1
  MotorDirections/1 -> motors_cmdout/1
  ThrustToMotorCommand/1 -> Saturation5/1
  thrusts_refin/1 -> ThrustToMotorCommand/1

== system asbQuadcopters_SiFi/Sensor/Sensor System/Camera ==
  states : Inport
  Add1 : Sum
  Bus Selector1 : BusSelector  OutputSignals=V_ned
  Bus Selector3 : BusSelector  OutputSignals=X_ned
  Bus Selector4 : BusSelector  OutputSignals=Omega_body
  Data Type Conversion : DataTypeConversion  OutDataTypeStr=single
  Demux4 : Demux  Outputs=2
  Gain1 : Gain  Gain=0.8*[-1,1]
  Gain2 : Gain  Gain=-1
  Mux7 : Mux  Inputs=2
  Mux8 : Mux  Inputs=2
  Product : Product
  Product1 : Product
  Reshape : Reshape
  Select dx,dy : Selector  InputPortWidth=3  IndexOptions=Index vector (dialog)  Indices=[1 2]  OutputSizes=1
  Select dx,dy1 : Selector  InputPortWidth=3  IndexOptions=Index vector (dialog)  Indices=[1 2]  OutputSizes=1
  Select dz : Selector  InputPortWidth=3  IndexOptions=Index vector (dialog)  Indices=3  OutputSizes=1
  Select dz1 : Selector  InputPortWidth=3  IndexOptions=Index vector (dialog)  Indices=3  OutputSizes=1
  SwitchPlanarOpticalFlow : Selector  InputPortWidth=2  IndexOptions=Index vector (dialog)  Indices=[2 1]  OutputSizes=1
  VelocityToOpticalFlow_Gain : Gain  Gain=Sensors.velocityToOpticalFlowGain
  opticalFlow_datout : Outport
  wires:
  Gain1/1 -> Demux4/1
  Data Type Conversion/1 -> opticalFlow_datout/1
  Bus Selector4/1 -> Reshape/1  "<Omega_body>"
  Select dz1/1 -> Gain2/1
  Bus Selector3/1 -> Select dz1/1  "<X_ned>"
  Select dz/1 -> Mux8/2
  Gain2/1 -> Product1/2, Product/2
  Mux8/1 -> VelocityToOpticalFlow_Gain/1
  Demux4/1 -> Product/1
  states/1 -> Bus Selector1/1, Bus Selector4/1, Bus Selector3/1
  Add1/1 -> Mux8/1
  Product/1 -> Mux7/1
  Product1/1 -> Mux7/2
  Demux4/2 -> Product1/1
  Bus Selector1/1 -> Select dz/1, Select dx,dy/1  "<V_ned>"
  Reshape/1 -> Select dx,dy1/1
  Select dx,dy1/1 -> Gain1/1
  Select dx,dy/1 -> Add1/1
  Mux7/1 -> SwitchPlanarOpticalFlow/1
  VelocityToOpticalFlow_Gain/1 -> Data Type Conversion/1
  SwitchPlanarOpticalFlow/1 -> Add1/2

== system asbQuadcopters_SiFi/Sensor/Sensor System/IMU_Pressure ==
  States : Inport
  Environment : Inport  Port=2
  Assumes takeoff was level1 : Bias  Bias=Sensors.altToPrsBias
  Bus Selector : BusSelector  OutputSignals=Accel_body,Omega_body,dOmega_body,DCM_be,X_ned
  Bus Selector1 : BusSelector  OutputSignals=Gravity_ned
  CG location : Constant  Value=Sensors.IMU.cg
  Data Type Conversion{,1..4} (5 alike) : DataTypeConversion  OutDataTypeStr=single
  Demux : Demux  Outputs=3
  Demux2 : Demux  Outputs=3
  HAL_acquisition_creator : Subsystem
  Mux : Mux  Inputs=8
  Product : Product  Multiplication=Matrix(*)
  Saturation : Saturate  UpperLimit=inf  LowerLimit=Sensors.altSensorMin  OutDataTypeStr=single
  Selector2 : Selector  InputPortWidth=3  IndexOptions=Index vector (dialog)  Indices=[3]  OutputSizes=1
  Three-axis Inertial Measurement Unit : aerolibnav/Three-axis Inertial Measurement Unit  units=Metric (MKS)  imu=Sensors.IMU.location  i_Ts=Ts  dtype_a=off  w_a=.7  z_a=.2  a_sf_cc=Sensors.IMU.accScaleCross  a_bias=Sensors.IMU.accBias  a_sat=Sensors.IMU.accLimits  dtype_g=off  w_g=.7  z_g=.2  g_sf_cc=Sensors.IMU.gyroScaleCross  g_bias=Sensors.IMU.gyroBias  g_sens=Sensors.IMU.gyroGBias  g_sat=Sensors.IMU.gyroLimits  i_rand=on  i_seeds=Sensors.IMU.noiseSeeds  i_pow=Sensors.IMU.noisePower
  altToprs_gain : Gain  Gain=Sensors.altToPrsGain  ParamDataTypeStr=single  OutDataTypeStr=single
  altToprs_gain1 : Gain  Gain=-1  ParamDataTypeStr=single  OutDataTypeStr=single
  sensordata_datout : Outport  OutDataTypeStr=Bus: HAL_acquisition_t
  wires:
  altToprs_gain/1 -> Assumes takeoff was level1/1  "prs"
  Demux/3 -> Mux/3  "ddz"
  Demux2/3 -> Mux/6  "r"
  Demux2/1 -> Mux/4  "p"
  Data Type Conversion1/1 -> HAL_acquisition_creator/1(sensors)
  Demux/1 -> Mux/1  "ddx"
  Data Type Conversion2/1 -> Demux2/1
  Three-axis Inertial Measurement Unit/2 -> Data Type Conversion2/1
  Demux/2 -> Mux/2  "ddy"
  Saturation/1 -> Data Type Conversion3/1  "altitude_sonar"
  Environment/1 -> Bus Selector1/1
  CG location/1 -> Three-axis Inertial Measurement Unit/4
  HAL_acquisition_creator/1(HAL_acquisition_t) -> sensordata_datout/1
  Bus Selector/1 -> Three-axis Inertial Measurement Unit/1  "<Accel_body>"
  altToprs_gain1/1 -> Saturation/1
  Bus Selector/3 -> Three-axis Inertial Measurement Unit/3  "<dOmega_body>"
  Bus Selector1/1 -> Product/2  "<Gravity_ned>"
  Bus Selector/4 -> Product/1  "<DCM_be>"
  Data Type Conversion3/1 -> Mux/7
  Bus Selector/2 -> Three-axis Inertial Measurement Unit/2  "<Omega_body>"
  Assumes takeoff was level1/1 -> Data Type Conversion4/1
  Product/1 -> Three-axis Inertial Measurement Unit/5
  Mux/1 -> Data Type Conversion1/1
  Data Type Conversion/1 -> Demux/1
  Data Type Conversion4/1 -> Mux/8
  States/1 -> Bus Selector/1
  Selector2/1 -> altToprs_gain/1, altToprs_gain1/1
  Bus Selector/5 -> Selector2/1  "<X_ned>"
  Demux2/2 -> Mux/5  "q"
  Three-axis Inertial Measurement Unit/1 -> Data Type Conversion/1

== system asbQuadcopters_SiFi/Airframe/AC model/Drag Calculation/Drag Calc ==
  Density : Inport  Unit=kg/m^3
  vel : Inport  Port=2  Unit=m/s
  Dynamic Pressure : aerolibasang/Dynamic Pressure
  FAULT_Dynamic Pressure : F_Line_block/Subsystem
  FAULT_Dynamic Pressure_2 : F_Line_block/Subsystem
  Gain : Gain  Gain=[.25 .25]
  FAULT_Gain : F_Line_block/Subsystem
  Mux1 : Mux  Inputs=2
  FAULT_Mux1 : F_Line_block/Subsystem
  FAULT_Mux1_2 : F_Line_block/Subsystem
  Product : Product  Inputs=3  RndMeth=Zero
  FAULT_Product : F_Line_block/Subsystem
  FAULT_Product_2 : F_Line_block/Subsystem
  FAULT_Product_3 : F_Line_block/Subsystem
  diameter : Constant  Value=Vehicle.Airframe.diameter  SampleTime=0
  dragCoeff : Constant  Value=Vehicle.Airframe.Cdx  SampleTime=0
  drag : Outport  Unit=N
  FAULT_drag : F_Line_block/Subsystem
  wires:
  Product/1 -> FAULT_drag/1
  FAULT_drag/1 -> drag/1
  dragCoeff/1 -> FAULT_Product_3/1  "Cd"
  FAULT_Product_3/1 -> Product/3
  Dynamic Pressure/1 -> FAULT_Product/1  "q"
  FAULT_Product/1 -> Product/1
  diameter/1 -> FAULT_Gain/1, FAULT_Mux1_2/1
  FAULT_Gain/1 -> Gain/1
  FAULT_Mux1_2/1 -> Mux1/2
  Mux1/1 -> FAULT_Product_2/1  "S"
  FAULT_Product_2/1 -> Product/2
  Gain/1 -> FAULT_Mux1/1
  FAULT_Mux1/1 -> Mux1/1
  vel/1 -> FAULT_Dynamic Pressure/1
  FAULT_Dynamic Pressure/1 -> Dynamic Pressure/1
  Density/1 -> FAULT_Dynamic Pressure_2/1
  FAULT_Dynamic Pressure_2/1 -> Dynamic Pressure/2

== system asbQuadcopters_SiFi/Airframe/AC model/Motor Forces and Torques/For Each Subsystem ==
  Vb : Inport  PortDimensions=3
  rho : Inport  Port=2  PortDimensions=1
  Omega : Inport  Port=3
  w : Inport  Port=4  Partition=on  PartitionDimension=2  PartitionWidth=1  PartitionOffset=0
  D : Inport  Port=5  Partition=on  PartitionDimension=2  PartitionWidth=1  PartitionOffset=0
  For Each : ForEach  DisableCoverage=on  IndexMode=One-based
  FAULT_For Each : F_Line_block/Subsystem
  Subsystem : Subsystem
  Forces : Outport  ConcatenationDimension=2
  FAULT_Forces : F_Line_block/Subsystem
  Moments : Outport  Port=2  ConcatenationDimension=2
  FAULT_Moments : F_Line_block/Subsystem
  wires:
  Vb/1 -> Subsystem/1(Vb)
  Omega/1 -> Subsystem/2(pqr)
  rho/1 -> Subsystem/3(rho)
  w/1 -> Subsystem/4(w)
  D/1 -> Subsystem/5(Arm)
  Subsystem/1(Fxyz) -> FAULT_Forces/1
  FAULT_Forces/1 -> Forces/1
  Subsystem/2(Mxyz) -> FAULT_Moments/1
  FAULT_Moments/1 -> Moments/1

== system asbQuadcopters_SiFi/Airframe/AC model/Motor Forces and Torques/MotorsToW ==
  motors_datin : Inport
  Motordirections : Gain  Gain=[1 -1 1 -1]  ParamDataTypeStr=single  OutDataTypeStr=Inherit: Inherit via back propagation  SaturateOnIntegerOverflow=on
  FAULT_Motordirections : F_Line_block/Subsystem
  Motordirections1 : Gain  Gain=[1 -1 1 -1]  ParamDataTypeStr=single  OutDataTypeStr=Inherit: Inherit via back propagation  SaturateOnIntegerOverflow=on
  FAULT_Motordirections1 : F_Line_block/Subsystem
  Saturation5 : Saturate  UpperLimit=Vehicle.Motor.maxLimit  LowerLimit=Vehicle.Motor.minLimit  OutDataTypeStr=Inherit: Inherit via back propagation
  FAULT_Saturation5 : F_Line_block/Subsystem
  Signed Sqrt : Sqrt  Operator=signedSqrt  OutDataTypeStr=Inherit: Inherit via back propagation  SaturateOnIntegerOverflow=on
  FAULT_Signed Sqrt : F_Line_block/Subsystem
  motorsToW2_Gain : Gain  Gain=Vehicle.Motor.commandToW2Gain  ParamDataTypeStr=single  OutDataTypeStr=Inherit: Inherit via back propagation  SaturateOnIntegerOverflow=on
  FAULT_motorsToW2_Gain : F_Line_block/Subsystem
  omegas_datout : Outport
  FAULT_omegas_datout : F_Line_block/Subsystem
  wires:
  motorsToW2_Gain/1 -> FAULT_Signed Sqrt/1
  FAULT_Signed Sqrt/1 -> Signed Sqrt/1
  Motordirections/1 -> FAULT_Saturation5/1
  FAULT_Saturation5/1 -> Saturation5/1
  Saturation5/1 -> FAULT_Motordirections1/1
  FAULT_Motordirections1/1 -> Motordirections1/1
  Motordirections1/1 -> FAULT_motorsToW2_Gain/1
  FAULT_motorsToW2_Gain/1 -> motorsToW2_Gain/1
  Signed Sqrt/1 -> FAULT_omegas_datout/1
  FAULT_omegas_datout/1 -> omegas_datout/1
  motors_datin/1 -> FAULT_Motordirections/1
  FAULT_Motordirections/1 -> Motordirections/1

== system asbQuadcopters_SiFi/FCS/State Estimator/Complementary Filter/If Action Subsystem ==
  rpy : Inport
  accel : Inport  Port=2
  Action Port : ActionPort  ActionType=then
  FAULT_Action Port : F_Line_block/Subsystem
  Demux : Demux  Outputs=3
  FAULT_Demux : F_Line_block/Subsystem
  Demux1 : Demux  Outputs=3
  FAULT_Demux1 : F_Line_block/Subsystem
  Divide : Product  Inputs=*/
  FAULT_Divide : F_Line_block/Subsystem
  FAULT_Divide_2 : F_Line_block/Subsystem
  Gain : Gain  Gain=1-Estimator.gyroAngleUpdateAccWeight
  FAULT_Gain{,1..4} (5 alike) : F_Line_block/Subsystem
  Gain1 : Gain  Gain=Estimator.gyroAngleUpdateAccWeight
  Gain2 : Gain  Gain=1/g
  Gain3 : Gain  Gain=Estimator.gyroAngleUpdateAccWeight
  Gain4 : Gain  Gain=1-Estimator.gyroAngleUpdateAccWeight
  Mux : Mux  Inputs=2
  FAULT_Mux : F_Line_block/Subsystem
  FAULT_Mux_2 : F_Line_block/Subsystem
  Sum : Sum  Inputs=|++
  FAULT_Sum : F_Line_block/Subsystem
  FAULT_Sum_2 : F_Line_block/Subsystem
  Sum1 : Sum  Inputs=|++
  FAULT_Sum1 : F_Line_block/Subsystem
  FAULT_Sum1_2 : F_Line_block/Subsystem
  Terminator1 : Terminator
  FAULT_Terminator1 : F_Line_block/Subsystem
  Trigonometric Function : Trigonometry  Operator=atan
  FAULT_Trigonometric Function : F_Line_block/Subsystem
  Trigonometric Function1 : Trigonometry  Operator=asin
  FAULT_Trigonometric Function1 : F_Line_block/Subsystem
  pitch,roll : Outport
  FAULT_pitch,roll : F_Line_block/Subsystem
  wires:
  accel/1 -> FAULT_Demux/1
  FAULT_Demux/1 -> Demux/1
  Demux/2 -> FAULT_Divide/1
  FAULT_Divide/1 -> Divide/1
  Demux/3 -> FAULT_Divide_2/1
  FAULT_Divide_2/1 -> Divide/2
  Divide/1 -> FAULT_Trigonometric Function/1
  FAULT_Trigonometric Function/1 -> Trigonometric Function/1
  Gain/1 -> FAULT_Sum/1
  FAULT_Sum/1 -> Sum/1
  Trigonometric Function/1 -> FAULT_Gain1/1
  FAULT_Gain1/1 -> Gain1/1
  Mux/1 -> FAULT_pitch,roll/1
  FAULT_pitch,roll/1 -> pitch,roll/1
  Gain2/1 -> FAULT_Trigonometric Function1/1
  FAULT_Trigonometric Function1/1 -> Trigonometric Function1/1
  Trigonometric Function1/1 -> FAULT_Gain3/1
  FAULT_Gain3/1 -> Gain3/1
  Gain4/1 -> FAULT_Sum1/1
  FAULT_Sum1/1 -> Sum1/1
  Gain3/1 -> FAULT_Sum1_2/1
  FAULT_Sum1_2/1 -> Sum1/2
  Sum1/1 -> FAULT_Mux/1
  FAULT_Mux/1 -> Mux/1
  Sum/1 -> FAULT_Mux_2/1
  FAULT_Mux_2/1 -> Mux/2
  rpy/1 -> FAULT_Demux1/1
  FAULT_Demux1/1 -> Demux1/1
  Demux1/1 -> FAULT_Gain/1
  FAULT_Gain/1 -> Gain/1
  Demux1/2 -> FAULT_Gain4/1
  FAULT_Gain4/1 -> Gain4/1
  Demux/1 -> FAULT_Gain2/1
  FAULT_Gain2/1 -> Gain2/1
  Demux1/3 -> FAULT_Terminator1/1
  FAULT_Terminator1/1 -> Terminator1/1
  Gain1/1 -> FAULT_Sum_2/1
  FAULT_Sum_2/1 -> Sum/2

== system asbQuadcopters_SiFi/FCS/State Estimator/Complementary Filter/If Action Subsystem1 ==
  rpy : Inport
  yawVis : Inport  Port=2
  Action Port : ActionPort  ActionType=then
  FAULT_Action Port : F_Line_block/Subsystem
  Gain : Gain  Gain=1-Estimator.gyroAngleUpdateVisWeight
  FAULT_Gain : F_Line_block/Subsystem
  Gain1 : Gain  Gain=Estimator.gyroAngleUpdateVisWeight
  FAULT_Gain1 : F_Line_block/Subsystem
  Selector4 : Selector  InputPortWidth=3  IndexOptions=Index vector (dialog)  Indices=[3]  OutputSizes=1
  FAULT_Selector4 : F_Line_block/Subsystem
  Sum : Sum  Inputs=|++
  FAULT_Sum : F_Line_block/Subsystem
  FAULT_Sum_2 : F_Line_block/Subsystem
  yaw : Outport
  FAULT_yaw : F_Line_block/Subsystem
  wires:
  rpy/1 -> FAULT_Selector4/1
  FAULT_Selector4/1 -> Selector4/1
  Selector4/1 -> FAULT_Gain/1
  FAULT_Gain/1 -> Gain/1
  yawVis/1 -> FAULT_Gain1/1
  FAULT_Gain1/1 -> Gain1/1
  Gain/1 -> FAULT_Sum/1
  FAULT_Sum/1 -> Sum/1
  Gain1/1 -> FAULT_Sum_2/1
  FAULT_Sum_2/1 -> Sum/2
  Sum/1 -> FAULT_yaw/1
  FAULT_yaw/1 -> yaw/1

== system asbQuadcopters_SiFi/FCS/State Estimator/Complementary Filter/If Action Subsystem2 ==
  prin : Inport
  Action Port : ActionPort  ActionType=else
  FAULT_Action Port : F_Line_block/Subsystem
  prout : Outport
  FAULT_prout : F_Line_block/Subsystem
  wires:
  prin/1 -> FAULT_prout/1
  FAULT_prout/1 -> prout/1

== system asbQuadcopters_SiFi/FCS/State Estimator/Complementary Filter/If Action Subsystem3 ==
  yawin : Inport
  Action Port : ActionPort  ActionType=else
  FAULT_Action Port : F_Line_block/Subsystem
  yout : Outport
  FAULT_yout : F_Line_block/Subsystem
  wires:
  yawin/1 -> FAULT_yout/1
  FAULT_yout/1 -> yout/1
